simulink model "Model_M4"  (R2018a)
settings: Solver=VariableStepAuto  StartTime=0.0  StopTime=1  RelTol=1e-3
libraries: simulink x3
settings Model: Creator=Aniket Raj  LastModifiedBy=Aniket Raj

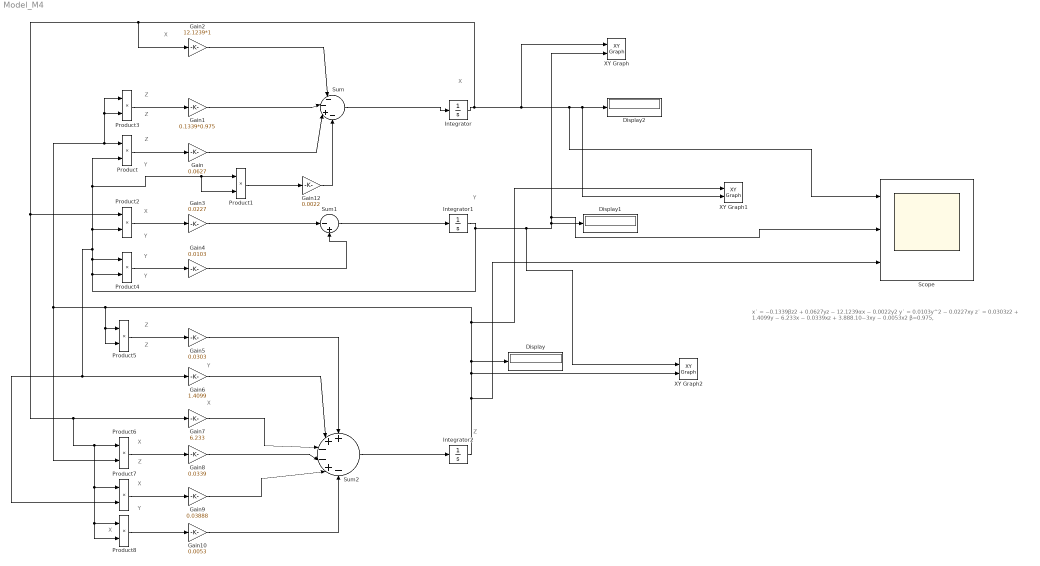
== system Model_M4 ==
  note: x˙ = −0.1339βz2 + 0.0627yz − 12.1239αx − 0.0022y2
      | y˙ = 0.0103y^2 − 0.0227xy
      | z˙ = 0.0303z2 + 1.4099y − 6.233x − 0.0339xz + 3.888.10−3xy − 0.0053x2
      |
      | β=0.975,
  note: Z
  note: Z
  note: X
  note: Y
  note: Z
  note: X
  note: X
  note: X
  note: Y
  note: X
  note: Z
  note: Y
  note: Z
  note: Y
  note: Y
  note: Z
  note: Z
  note: X
  note: Y
  note: Y
  note: X
  Display : Display
  Display1 : Display
  Display2 : Display
  Gain : Gain  Gain=0.0627
  Gain1 : Gain  Gain=0.1339*0.975
  Gain10 : Gain  Gain=0.0053
  Gain12 : Gain  Gain=0.0022
  Gain2 : Gain  Gain=12.1239*1
  Gain3 : Gain  Gain=0.0227
  Gain4 : Gain  Gain=0.0103
  Gain5 : Gain  Gain=0.0303
  Gain6 : Gain  Gain=1.4099
  Gain7 : Gain  Gain=6.233
  Gain8 : Gain  Gain=0.0339
  Gain9 : Gain  Gain=0.03888
  Integrator : Integrator  InitialCondition=161.3367
  Integrator1 : Integrator  InitialCondition=807.6816
  Integrator2 : Integrator  InitialCondition=204.2714
  Product{,1..8} (9 alike) : Product
  Scope : Scope  NumInputPorts=3
  Sum : Sum  Inputs=|-|-|+|-
  Sum1 : Sum  Inputs=|-+
  Sum2 : Sum  Inputs=+|+|-|-|+|-
  XY Graph : simulink/Sinks/XY Graph  xmin=-50000  xmax=50000  ymin=-50000  ymax=50000  st=0.01
  XY Graph1 : simulink/Sinks/XY Graph  xmin=-50000  xmax=50000  ymin=-50000  ymax=50000  st=0.01
  XY Graph2 : simulink/Sinks/XY Graph  xmin=-50000  xmax=50000  ymin=-50000  ymax=50000  st=0.01
  wires:
  Integrator1/1 -> XY Graph2/1, Scope/2, XY Graph/2, Display1/1, Product4/1, Product7/2, Gain6/1, Product2/2, Product1/2, Product1/1, Product/2, Product4/2
  Product7/1 -> Gain9/1
  Gain3/1 -> Sum1/1
  Gain8/1 -> Sum2/4
  Product5/1 -> Gain5/1
  Gain7/1 -> Sum2/3
  Gain10/1 -> Sum2/6
  Integrator/1 -> XY Graph/1, Scope/1, XY Graph1/2, Display2/1, Gain2/1, Product8/2, Product8/1, Product7/1, Product6/1, Gain7/1, Product2/1
  Product8/1 -> Gain10/1
  Gain9/1 -> Sum2/5
  Gain5/1 -> Sum2/1
  Product2/1 -> Gain3/1
  Product3/1 -> Gain1/1
  Integrator2/1 -> Scope/3, XY Graph2/2, Display/1, XY Graph1/1, Product3/1, Product3/2, Product/1, Product6/2, Product5/2, Product5/1
  Sum/1 -> Integrator/1
  Gain2/1 -> Sum/1
  Gain1/1 -> Sum/2
  Product/1 -> Gain/1
  Sum2/1 -> Integrator2/1
  Product4/1 -> Gain4/1
  Product6/1 -> Gain8/1
  Sum1/1 -> Integrator1/1
  Gain4/1 -> Sum1/2
  Gain/1 -> Sum/3
  Gain6/1 -> Sum2/2
  Product1/1 -> Gain12/1
  Gain12/1 -> Sum/4
